simulink model "fuzzy_controller_5_gauss"  (R2016a)
settings: Solver=ode45  StartTime=0.0  StopTime=10.0  RelTol=1e-3
values from neighbouring files (symbols this model uses):
  FORCE_Range_1 = -150    [fuzzy_controller_3_trimf_params.m]    (also in fuzzy_controller_5_gauss_params.m; fuzzy_controller_5_gbell_params.m; fuzzy_controller_5_trimf_optimal_params.m; fuzzy_controller_5_trimf_params.m)
  FORCE_Range_2 = 150    [fuzzy_controller_3_trimf_params.m]    (also in fuzzy_controller_5_gauss_params.m; fuzzy_controller_5_gbell_params.m; fuzzy_controller_5_trimf_optimal_params.m; fuzzy_controller_5_trimf_params.m)
undefined symbols (not defined in the file): fi_1_mu, fi_1_sigma, fi_2_mu, fi_2_sigma, fi_3_mu, fi_3_sigma, fi_4_mu, fi_4_sigma, fi_5_mu, fi_5_sigma, force_1_mu, force_1_sigma, force_2_mu, force_2_sigma, force_3_mu, force_3_sigma, force_4_mu, force_4_sigma, force_5_mu, force_5_sigma, omega_1_mu, omega_1_sigma, omega_2_mu, omega_2_sigma, omega_3_mu, omega_3_sigma, omega_4_mu, omega_4_sigma, omega_5_mu, omega_5_sigma
libraries: fuzwiz x2
settings Model: Creator=Руслан  LastModifiedBy=Руслан
settings DataIOCC: LimitDataPoints=on  SaveFormat=Array
settings DebuggingCC: AlgebraicLoopMsg=error
settings HardwareCC: ProdBitPerLong=64  ProdLargestAtomicFloat=None  ProdHWDeviceType=Intel->x86-64
settings ModelReferenceCC: PropagateSignalLabelsOutOfModel=off
settings RTWCC: TemplateMakefile=RTW.MSVCBuild  Description=Create Visual C/C++ Solution File for Simulink Coder  GenerateReport=on  RetainRTWFile=on  LaunchReport=on
settings CodeAppCC: ForceParamTrailComments=on  MATLABSourceComments=on
settings GRTTargetCC: TargetLangStandard=C99 (ISO)
settings ConfigComp: CovModelRefEnable=Off

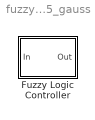
== system fuzzy_controller_5_gauss ==
  Fuzzy Logic Controller : Subsystem

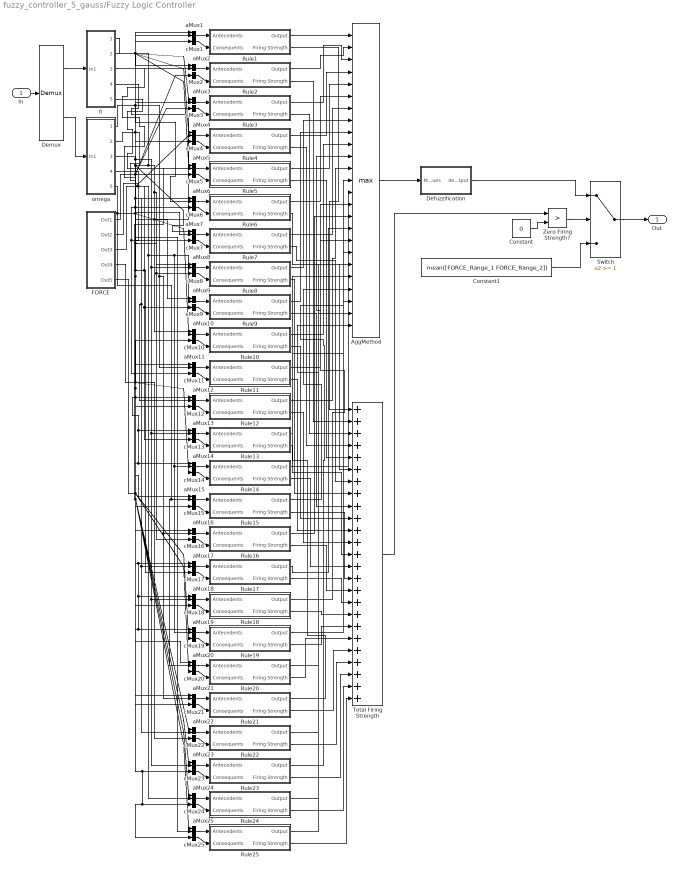
== system fuzzy_controller_5_gauss/Fuzzy Logic Controller ==
  In : Inport
  AggMethod : MinMax  Function=max  Inputs=25
  Constant : Constant  Value=0
  Constant1 : Constant  Value=mean([FORCE_Range_1 FORCE_Range_2])
  Defuzzification : Subsystem
  Demux : Demux  Outputs=2
  FORCE : Subsystem
  Rule1 : Subsystem
  Rule10 : Subsystem
  Rule11 : Subsystem
  Rule12 : Subsystem
  Rule13 : Subsystem
  Rule14 : Subsystem
  Rule15 : Subsystem
  Rule16 : Subsystem
  Rule17 : Subsystem
  Rule18 : Subsystem
  Rule19 : Subsystem
  Rule2 : Subsystem
  Rule20 : Subsystem
  Rule21 : Subsystem
  Rule22 : Subsystem
  Rule23 : Subsystem
  Rule24 : Subsystem
  Rule25 : Subsystem
  Rule3 : Subsystem
  Rule4 : Subsystem
  Rule5 : Subsystem
  Rule6 : Subsystem
  Rule7 : Subsystem
  Rule8 : Subsystem
  Rule9 : Subsystem
  Switch : Switch  Threshold=1
  Total Firing Strength : Sum  Inputs=25
  Zero Firing Strength? : RelationalOperator  Operator=>  OutDataTypeStr=boolean
  aMux{1..25} (25 alike) : Mux  Inputs=2
  cMux{1..25} (25 alike) : Mux  Inputs=1
  fi : Subsystem
  omega : Subsystem
  Out : Outport
  wires:
  Rule1/1(Output) -> AggMethod/1
  Rule2/1(Output) -> AggMethod/2
  Rule5/1(Output) -> AggMethod/5
  Rule4/1(Output) -> AggMethod/4
  Rule3/1(Output) -> AggMethod/3
  Rule1/2(Firing Strength) -> Total Firing Strength/1
  Rule2/2(Firing Strength) -> Total Firing Strength/2
  Rule3/2(Firing Strength) -> Total Firing Strength/3
  Rule4/2(Firing Strength) -> Total Firing Strength/4
  Rule5/2(Firing Strength) -> Total Firing Strength/5
  Total Firing Strength/1 -> Zero Firing Strength?/1
  Constant/1 -> Zero Firing Strength?/2
  Zero Firing Strength?/1 -> Switch/2
  Switch/1 -> Out/1
  Constant1/1 -> Switch/3
  AggMethod/1 -> Defuzzification/1(MF values)
  Defuzzification/1(defuzzified output) -> Switch/1
  Demux/1 -> fi/1(In1)
  In/1 -> Demux/1
  Demux/2 -> omega/1(In1)
  Rule9/2(Firing Strength) -> Total Firing Strength/9
  Rule8/2(Firing Strength) -> Total Firing Strength/8
  Rule7/2(Firing Strength) -> Total Firing Strength/7
  Rule6/2(Firing Strength) -> Total Firing Strength/6
  Rule9/1(Output) -> AggMethod/9
  Rule8/1(Output) -> AggMethod/8
  Rule7/1(Output) -> AggMethod/7
  Rule6/1(Output) -> AggMethod/6
  aMux9/1 -> Rule9/1(Antecedents)
  aMux8/1 -> Rule8/1(Antecedents)
  aMux7/1 -> Rule7/1(Antecedents)
  aMux6/1 -> Rule6/1(Antecedents)
  aMux5/1 -> Rule5/1(Antecedents)
  aMux4/1 -> Rule4/1(Antecedents)
  aMux3/1 -> Rule3/1(Antecedents)
  aMux2/1 -> Rule2/1(Antecedents)
  aMux1/1 -> Rule1/1(Antecedents)
  aMux10/1 -> Rule10/1(Antecedents)
  aMux11/1 -> Rule11/1(Antecedents)
  aMux12/1 -> Rule12/1(Antecedents)
  aMux13/1 -> Rule13/1(Antecedents)
  aMux14/1 -> Rule14/1(Antecedents)
  aMux15/1 -> Rule15/1(Antecedents)
  aMux16/1 -> Rule16/1(Antecedents)
  aMux17/1 -> Rule17/1(Antecedents)
  aMux18/1 -> Rule18/1(Antecedents)
  aMux19/1 -> Rule19/1(Antecedents)
  aMux25/1 -> Rule25/1(Antecedents)
  aMux24/1 -> Rule24/1(Antecedents)
  aMux23/1 -> Rule23/1(Antecedents)
  aMux22/1 -> Rule22/1(Antecedents)
  aMux21/1 -> Rule21/1(Antecedents)
  aMux20/1 -> Rule20/1(Antecedents)
  Rule25/2(Firing Strength) -> Total Firing Strength/25
  Rule10/2(Firing Strength) -> Total Firing Strength/10
  Rule11/2(Firing Strength) -> Total Firing Strength/11
  Rule12/2(Firing Strength) -> Total Firing Strength/12
  Rule13/2(Firing Strength) -> Total Firing Strength/13
  Rule14/2(Firing Strength) -> Total Firing Strength/14
  Rule15/2(Firing Strength) -> Total Firing Strength/15
  Rule16/2(Firing Strength) -> Total Firing Strength/16
  Rule17/2(Firing Strength) -> Total Firing Strength/17
  Rule18/2(Firing Strength) -> Total Firing Strength/18
  Rule19/2(Firing Strength) -> Total Firing Strength/19
  Rule20/2(Firing Strength) -> Total Firing Strength/20
  Rule21/2(Firing Strength) -> Total Firing Strength/21
  Rule22/2(Firing Strength) -> Total Firing Strength/22
  Rule23/2(Firing Strength) -> Total Firing Strength/23
  Rule24/2(Firing Strength) -> Total Firing Strength/24
  Rule10/1(Output) -> AggMethod/10
  Rule11/1(Output) -> AggMethod/11
  Rule12/1(Output) -> AggMethod/12
  Rule13/1(Output) -> AggMethod/13
  Rule14/1(Output) -> AggMethod/14
  Rule15/1(Output) -> AggMethod/15
  Rule16/1(Output) -> AggMethod/16
  Rule25/1(Output) -> AggMethod/25
  Rule17/1(Output) -> AggMethod/17
  Rule18/1(Output) -> AggMethod/18
  Rule19/1(Output) -> AggMethod/19
  Rule20/1(Output) -> AggMethod/20
  Rule21/1(Output) -> AggMethod/21
  Rule22/1(Output) -> AggMethod/22
  Rule23/1(Output) -> AggMethod/23
  Rule24/1(Output) -> AggMethod/24
  cMux1/1 -> Rule1/2(Consequents)
  fi/1(Out1) -> aMux1/1, aMux2/1, aMux3/1, aMux4/1, aMux5/1
  omega/1(Out1) -> aMux16/2, aMux21/2, aMux11/2, aMux1/2, aMux6/2
  FORCE/1(Out1) -> cMux7/1, cMux11/1, cMux6/1, cMux1/1, cMux2/1, cMux3/1
  cMux2/1 -> Rule2/2(Consequents)
  omega/2(Out2) -> aMux7/2, aMux12/2, aMux17/2, aMux22/2, aMux2/2
  cMux3/1 -> Rule3/2(Consequents)
  omega/3(Out3) -> aMux23/2, aMux18/2, aMux13/2, aMux8/2, aMux3/2
  cMux4/1 -> Rule4/2(Consequents)
  omega/4(Out4) -> aMux14/2, aMux19/2, aMux9/2, aMux24/2, aMux4/2
  FORCE/2(Out2) -> cMux8/1, cMux16/1, cMux4/1, cMux12/1
  cMux5/1 -> Rule5/2(Consequents)
  omega/5(Out5) -> aMux5/2, aMux10/2, aMux25/2, aMux20/2, aMux15/2
  FORCE/3(Out3) -> cMux5/1, cMux21/1, cMux17/1, cMux9/1, cMux13/1
  cMux6/1 -> Rule6/2(Consequents)
  fi/2(Out2) -> aMux8/1, aMux9/1, aMux10/1, aMux6/1, aMux7/1
  cMux7/1 -> Rule7/2(Consequents)
  cMux8/1 -> Rule8/2(Consequents)
  cMux9/1 -> Rule9/2(Consequents)
  cMux10/1 -> Rule10/2(Consequents)
  FORCE/4(Out4) -> cMux10/1, cMux14/1, cMux18/1, cMux22/1
  cMux11/1 -> Rule11/2(Consequents)
  fi/3(Out3) -> aMux15/1, aMux14/1, aMux13/1, aMux12/1, aMux11/1
  cMux12/1 -> Rule12/2(Consequents)
  cMux13/1 -> Rule13/2(Consequents)
  cMux14/1 -> Rule14/2(Consequents)
  cMux15/1 -> Rule15/2(Consequents)
  FORCE/5(Out5) -> cMux25/1, cMux24/1, cMux23/1, cMux15/1, cMux19/1, cMux20/1
  cMux16/1 -> Rule16/2(Consequents)
  fi/4(Out4) -> aMux20/1, aMux19/1, aMux18/1, aMux17/1, aMux16/1
  cMux17/1 -> Rule17/2(Consequents)
  cMux18/1 -> Rule18/2(Consequents)
  cMux19/1 -> Rule19/2(Consequents)
  cMux20/1 -> Rule20/2(Consequents)
  cMux21/1 -> Rule21/2(Consequents)
  fi/5(Out5) -> aMux21/1, aMux22/1, aMux23/1, aMux24/1, aMux25/1
  cMux22/1 -> Rule22/2(Consequents)
  cMux23/1 -> Rule23/2(Consequents)
  cMux24/1 -> Rule24/2(Consequents)
  cMux25/1 -> Rule25/2(Consequents)

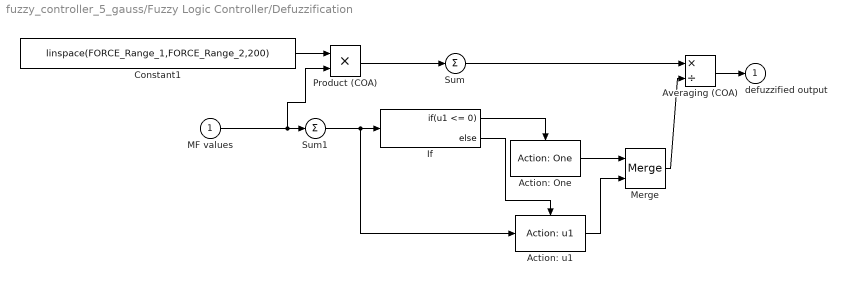
== system fuzzy_controller_5_gauss/Fuzzy Logic Controller/Defuzzification ==
  MF values : Inport
  Action: One : fuzwiz/Centroid of Area/Action: One
  Action: u1 : fuzwiz/Centroid of Area/Action: u1
  Averaging (COA) : Product  Inputs=*/  SaturateOnIntegerOverflow=on  RndMeth=Zero  InputSameDT=on  OutDataTypeStr=Inherit: Same as first input
  Constant1 : Constant  Value=linspace(FORCE_Range_1,FORCE_Range_2,200)
  If : If  IfExpression=u1 <= 0
  Merge : Merge
  Product (COA) : Product  SaturateOnIntegerOverflow=on  RndMeth=Zero  InputSameDT=on  OutDataTypeStr=Inherit: Same as first input
  Sum : Sum  Inputs=+  SaturateOnIntegerOverflow=on  InputSameDT=on  OutDataTypeStr=Inherit: Same as first input
  Sum1 : Sum  Inputs=+  SaturateOnIntegerOverflow=on  InputSameDT=on  OutDataTypeStr=Inherit: Same as first input
  defuzzified output : Outport
  wires:
  Merge/1 -> Averaging (COA)/2
  Action: u1/1 -> Merge/2
  Action: One/1 -> Merge/1
  If/1 -> Action: One/Action
  If/2 -> Action: u1/Action
  Sum1/1 -> Action: u1/1, If/1
  Constant1/1 -> Product (COA)/1
  Product (COA)/1 -> Sum/1
  MF values/1 -> Product (COA)/2, Sum1/1
  Sum/1 -> Averaging (COA)/1
  Averaging (COA)/1 -> defuzzified output/1

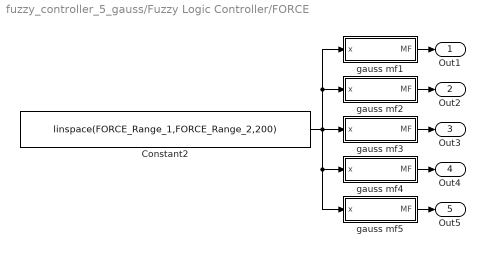
== system fuzzy_controller_5_gauss/Fuzzy Logic Controller/FORCE ==
  Constant2 : Constant  Value=linspace(FORCE_Range_1,FORCE_Range_2,200)
  gauss mf1 : Subsystem  mask{sigma=force_1_sigma, mu=force_1_mu}
      mask prompts: sigma "Variance sigma:"; mu "Mean c:"
  gauss mf2 : Subsystem  mask{sigma=force_2_sigma, mu=force_2_mu}
      mask prompts: sigma "Variance sigma:"; mu "Mean c:"
  gauss mf3 : Subsystem  mask{sigma=force_3_sigma, mu=force_3_mu}
      mask prompts: sigma "Variance sigma:"; mu "Mean c:"
  gauss mf4 : Subsystem  mask{sigma=force_4_sigma, mu=force_4_mu}
      mask prompts: sigma "Variance sigma:"; mu "Mean c:"
  gauss mf5 : Subsystem  mask{sigma=force_5_sigma, mu=force_5_mu}
      mask prompts: sigma "Variance sigma:"; mu "Mean c:"
  Out1 : Outport
  Out2 : Outport  Port=2
  Out3 : Outport  Port=3
  Out4 : Outport  Port=4
  Out5 : Outport  Port=5
  wires:
  Constant2/1 -> gauss mf3/1(x), gauss mf5/1(x), gauss mf4/1(x), gauss mf2/1(x), gauss mf1/1(x)
  gauss mf1/1(MF) -> Out1/1
  gauss mf2/1(MF) -> Out2/1
  gauss mf3/1(MF) -> Out3/1
  gauss mf4/1(MF) -> Out4/1
  gauss mf5/1(MF) -> Out5/1

== system fuzzy_controller_5_gauss/Fuzzy Logic Controller/Rule1 ==
  Antecedents : Inport
  Consequents : Inport  Port=2
  Weight : Constant
  Weighting : Product  SaturateOnIntegerOverflow=on  RndMeth=Zero  InputSameDT=on  OutDataTypeStr=Inherit: Same as first input
  andorMethod : MinMax  SaturateOnIntegerOverflow=on  InputSameDT=on
  impMethod : MinMax  Inputs=2  SaturateOnIntegerOverflow=on  InputSameDT=on
  Output : Outport
  Firing Strength : Outport  Port=2
  wires:
  impMethod/1 -> Output/1
  Weighting/1 -> Firing Strength/1, impMethod/1
  Consequents/1 -> impMethod/2
  Weight/1 -> Weighting/1
  andorMethod/1 -> Weighting/2
  Antecedents/1 -> andorMethod/1

== system fuzzy_controller_5_gauss/Fuzzy Logic Controller/Rule10 ==
  Antecedents : Inport
  Consequents : Inport  Port=2
  Weight : Constant
  Weighting : Product  SaturateOnIntegerOverflow=on  RndMeth=Zero  InputSameDT=on  OutDataTypeStr=Inherit: Same as first input
  andorMethod : MinMax  SaturateOnIntegerOverflow=on  InputSameDT=on
  impMethod : MinMax  Inputs=2  SaturateOnIntegerOverflow=on  InputSameDT=on
  Output : Outport
  Firing Strength : Outport  Port=2
  wires:
  impMethod/1 -> Output/1
  Weighting/1 -> Firing Strength/1, impMethod/1
  Consequents/1 -> impMethod/2
  Weight/1 -> Weighting/1
  andorMethod/1 -> Weighting/2
  Antecedents/1 -> andorMethod/1

== system fuzzy_controller_5_gauss/Fuzzy Logic Controller/Rule11 ==
  Antecedents : Inport
  Consequents : Inport  Port=2
  Weight : Constant
  Weighting : Product  SaturateOnIntegerOverflow=on  RndMeth=Zero  InputSameDT=on  OutDataTypeStr=Inherit: Same as first input
  andorMethod : MinMax  SaturateOnIntegerOverflow=on  InputSameDT=on
  impMethod : MinMax  Inputs=2  SaturateOnIntegerOverflow=on  InputSameDT=on
  Output : Outport
  Firing Strength : Outport  Port=2
  wires:
  impMethod/1 -> Output/1
  Weighting/1 -> Firing Strength/1, impMethod/1
  Consequents/1 -> impMethod/2
  Weight/1 -> Weighting/1
  andorMethod/1 -> Weighting/2
  Antecedents/1 -> andorMethod/1

== system fuzzy_controller_5_gauss/Fuzzy Logic Controller/Rule12 ==
  Antecedents : Inport
  Consequents : Inport  Port=2
  Weight : Constant
  Weighting : Product  SaturateOnIntegerOverflow=on  RndMeth=Zero  InputSameDT=on  OutDataTypeStr=Inherit: Same as first input
  andorMethod : MinMax  SaturateOnIntegerOverflow=on  InputSameDT=on
  impMethod : MinMax  Inputs=2  SaturateOnIntegerOverflow=on  InputSameDT=on
  Output : Outport
  Firing Strength : Outport  Port=2
  wires:
  impMethod/1 -> Output/1
  Weighting/1 -> Firing Strength/1, impMethod/1
  Consequents/1 -> impMethod/2
  Weight/1 -> Weighting/1
  andorMethod/1 -> Weighting/2
  Antecedents/1 -> andorMethod/1

== system fuzzy_controller_5_gauss/Fuzzy Logic Controller/Rule13 ==
  Antecedents : Inport
  Consequents : Inport  Port=2
  Weight : Constant
  Weighting : Product  SaturateOnIntegerOverflow=on  RndMeth=Zero  InputSameDT=on  OutDataTypeStr=Inherit: Same as first input
  andorMethod : MinMax  SaturateOnIntegerOverflow=on  InputSameDT=on
  impMethod : MinMax  Inputs=2  SaturateOnIntegerOverflow=on  InputSameDT=on
  Output : Outport
  Firing Strength : Outport  Port=2
  wires:
  impMethod/1 -> Output/1
  Weighting/1 -> Firing Strength/1, impMethod/1
  Consequents/1 -> impMethod/2
  Weight/1 -> Weighting/1
  andorMethod/1 -> Weighting/2
  Antecedents/1 -> andorMethod/1

== system fuzzy_controller_5_gauss/Fuzzy Logic Controller/Rule14 ==
  Antecedents : Inport
  Consequents : Inport  Port=2
  Weight : Constant
  Weighting : Product  SaturateOnIntegerOverflow=on  RndMeth=Zero  InputSameDT=on  OutDataTypeStr=Inherit: Same as first input
  andorMethod : MinMax  SaturateOnIntegerOverflow=on  InputSameDT=on
  impMethod : MinMax  Inputs=2  SaturateOnIntegerOverflow=on  InputSameDT=on
  Output : Outport
  Firing Strength : Outport  Port=2
  wires:
  impMethod/1 -> Output/1
  Weighting/1 -> Firing Strength/1, impMethod/1
  Consequents/1 -> impMethod/2
  Weight/1 -> Weighting/1
  andorMethod/1 -> Weighting/2
  Antecedents/1 -> andorMethod/1

== system fuzzy_controller_5_gauss/Fuzzy Logic Controller/Rule15 ==
  Antecedents : Inport
  Consequents : Inport  Port=2
  Weight : Constant
  Weighting : Product  SaturateOnIntegerOverflow=on  RndMeth=Zero  InputSameDT=on  OutDataTypeStr=Inherit: Same as first input
  andorMethod : MinMax  SaturateOnIntegerOverflow=on  InputSameDT=on
  impMethod : MinMax  Inputs=2  SaturateOnIntegerOverflow=on  InputSameDT=on
  Output : Outport
  Firing Strength : Outport  Port=2
  wires:
  impMethod/1 -> Output/1
  Weighting/1 -> Firing Strength/1, impMethod/1
  Consequents/1 -> impMethod/2
  Weight/1 -> Weighting/1
  andorMethod/1 -> Weighting/2
  Antecedents/1 -> andorMethod/1

== system fuzzy_controller_5_gauss/Fuzzy Logic Controller/Rule16 ==
  Antecedents : Inport
  Consequents : Inport  Port=2
  Weight : Constant
  Weighting : Product  SaturateOnIntegerOverflow=on  RndMeth=Zero  InputSameDT=on  OutDataTypeStr=Inherit: Same as first input
  andorMethod : MinMax  SaturateOnIntegerOverflow=on  InputSameDT=on
  impMethod : MinMax  Inputs=2  SaturateOnIntegerOverflow=on  InputSameDT=on
  Output : Outport
  Firing Strength : Outport  Port=2
  wires:
  impMethod/1 -> Output/1
  Weighting/1 -> Firing Strength/1, impMethod/1
  Consequents/1 -> impMethod/2
  Weight/1 -> Weighting/1
  andorMethod/1 -> Weighting/2
  Antecedents/1 -> andorMethod/1

== system fuzzy_controller_5_gauss/Fuzzy Logic Controller/Rule17 ==
  Antecedents : Inport
  Consequents : Inport  Port=2
  Weight : Constant
  Weighting : Product  SaturateOnIntegerOverflow=on  RndMeth=Zero  InputSameDT=on  OutDataTypeStr=Inherit: Same as first input
  andorMethod : MinMax  SaturateOnIntegerOverflow=on  InputSameDT=on
  impMethod : MinMax  Inputs=2  SaturateOnIntegerOverflow=on  InputSameDT=on
  Output : Outport
  Firing Strength : Outport  Port=2
  wires:
  impMethod/1 -> Output/1
  Weighting/1 -> Firing Strength/1, impMethod/1
  Consequents/1 -> impMethod/2
  Weight/1 -> Weighting/1
  andorMethod/1 -> Weighting/2
  Antecedents/1 -> andorMethod/1

== system fuzzy_controller_5_gauss/Fuzzy Logic Controller/Rule18 ==
  Antecedents : Inport
  Consequents : Inport  Port=2
  Weight : Constant
  Weighting : Product  SaturateOnIntegerOverflow=on  RndMeth=Zero  InputSameDT=on  OutDataTypeStr=Inherit: Same as first input
  andorMethod : MinMax  SaturateOnIntegerOverflow=on  InputSameDT=on
  impMethod : MinMax  Inputs=2  SaturateOnIntegerOverflow=on  InputSameDT=on
  Output : Outport
  Firing Strength : Outport  Port=2
  wires:
  impMethod/1 -> Output/1
  Weighting/1 -> Firing Strength/1, impMethod/1
  Consequents/1 -> impMethod/2
  Weight/1 -> Weighting/1
  andorMethod/1 -> Weighting/2
  Antecedents/1 -> andorMethod/1

== system fuzzy_controller_5_gauss/Fuzzy Logic Controller/Rule19 ==
  Antecedents : Inport
  Consequents : Inport  Port=2
  Weight : Constant
  Weighting : Product  SaturateOnIntegerOverflow=on  RndMeth=Zero  InputSameDT=on  OutDataTypeStr=Inherit: Same as first input
  andorMethod : MinMax  SaturateOnIntegerOverflow=on  InputSameDT=on
  impMethod : MinMax  Inputs=2  SaturateOnIntegerOverflow=on  InputSameDT=on
  Output : Outport
  Firing Strength : Outport  Port=2
  wires:
  impMethod/1 -> Output/1
  Weighting/1 -> Firing Strength/1, impMethod/1
  Consequents/1 -> impMethod/2
  Weight/1 -> Weighting/1
  andorMethod/1 -> Weighting/2
  Antecedents/1 -> andorMethod/1

== system fuzzy_controller_5_gauss/Fuzzy Logic Controller/Rule2 ==
  Antecedents : Inport
  Consequents : Inport  Port=2
  Weight : Constant
  Weighting : Product  SaturateOnIntegerOverflow=on  RndMeth=Zero  InputSameDT=on  OutDataTypeStr=Inherit: Same as first input
  andorMethod : MinMax  SaturateOnIntegerOverflow=on  InputSameDT=on
  impMethod : MinMax  Inputs=2  SaturateOnIntegerOverflow=on  InputSameDT=on
  Output : Outport
  Firing Strength : Outport  Port=2
  wires:
  impMethod/1 -> Output/1
  Weighting/1 -> Firing Strength/1, impMethod/1
  Consequents/1 -> impMethod/2
  Weight/1 -> Weighting/1
  andorMethod/1 -> Weighting/2
  Antecedents/1 -> andorMethod/1

== system fuzzy_controller_5_gauss/Fuzzy Logic Controller/Rule20 ==
  Antecedents : Inport
  Consequents : Inport  Port=2
  Weight : Constant
  Weighting : Product  SaturateOnIntegerOverflow=on  RndMeth=Zero  InputSameDT=on  OutDataTypeStr=Inherit: Same as first input
  andorMethod : MinMax  SaturateOnIntegerOverflow=on  InputSameDT=on
  impMethod : MinMax  Inputs=2  SaturateOnIntegerOverflow=on  InputSameDT=on
  Output : Outport
  Firing Strength : Outport  Port=2
  wires:
  impMethod/1 -> Output/1
  Weighting/1 -> Firing Strength/1, impMethod/1
  Consequents/1 -> impMethod/2
  Weight/1 -> Weighting/1
  andorMethod/1 -> Weighting/2
  Antecedents/1 -> andorMethod/1

== system fuzzy_controller_5_gauss/Fuzzy Logic Controller/Rule21 ==
  Antecedents : Inport
  Consequents : Inport  Port=2
  Weight : Constant
  Weighting : Product  SaturateOnIntegerOverflow=on  RndMeth=Zero  InputSameDT=on  OutDataTypeStr=Inherit: Same as first input
  andorMethod : MinMax  SaturateOnIntegerOverflow=on  InputSameDT=on
  impMethod : MinMax  Inputs=2  SaturateOnIntegerOverflow=on  InputSameDT=on
  Output : Outport
  Firing Strength : Outport  Port=2
  wires:
  impMethod/1 -> Output/1
  Weighting/1 -> Firing Strength/1, impMethod/1
  Consequents/1 -> impMethod/2
  Weight/1 -> Weighting/1
  andorMethod/1 -> Weighting/2
  Antecedents/1 -> andorMethod/1

== system fuzzy_controller_5_gauss/Fuzzy Logic Controller/Rule22 ==
  Antecedents : Inport
  Consequents : Inport  Port=2
  Weight : Constant
  Weighting : Product  SaturateOnIntegerOverflow=on  RndMeth=Zero  InputSameDT=on  OutDataTypeStr=Inherit: Same as first input
  andorMethod : MinMax  SaturateOnIntegerOverflow=on  InputSameDT=on
  impMethod : MinMax  Inputs=2  SaturateOnIntegerOverflow=on  InputSameDT=on
  Output : Outport
  Firing Strength : Outport  Port=2
  wires:
  impMethod/1 -> Output/1
  Weighting/1 -> Firing Strength/1, impMethod/1
  Consequents/1 -> impMethod/2
  Weight/1 -> Weighting/1
  andorMethod/1 -> Weighting/2
  Antecedents/1 -> andorMethod/1

== system fuzzy_controller_5_gauss/Fuzzy Logic Controller/Rule23 ==
  Antecedents : Inport
  Consequents : Inport  Port=2
  Weight : Constant
  Weighting : Product  SaturateOnIntegerOverflow=on  RndMeth=Zero  InputSameDT=on  OutDataTypeStr=Inherit: Same as first input
  andorMethod : MinMax  SaturateOnIntegerOverflow=on  InputSameDT=on
  impMethod : MinMax  Inputs=2  SaturateOnIntegerOverflow=on  InputSameDT=on
  Output : Outport
  Firing Strength : Outport  Port=2
  wires:
  impMethod/1 -> Output/1
  Weighting/1 -> Firing Strength/1, impMethod/1
  Consequents/1 -> impMethod/2
  Weight/1 -> Weighting/1
  andorMethod/1 -> Weighting/2
  Antecedents/1 -> andorMethod/1

== system fuzzy_controller_5_gauss/Fuzzy Logic Controller/Rule24 ==
  Antecedents : Inport
  Consequents : Inport  Port=2
  Weight : Constant
  Weighting : Product  SaturateOnIntegerOverflow=on  RndMeth=Zero  InputSameDT=on  OutDataTypeStr=Inherit: Same as first input
  andorMethod : MinMax  SaturateOnIntegerOverflow=on  InputSameDT=on
  impMethod : MinMax  Inputs=2  SaturateOnIntegerOverflow=on  InputSameDT=on
  Output : Outport
  Firing Strength : Outport  Port=2
  wires:
  impMethod/1 -> Output/1
  Weighting/1 -> Firing Strength/1, impMethod/1
  Consequents/1 -> impMethod/2
  Weight/1 -> Weighting/1
  andorMethod/1 -> Weighting/2
  Antecedents/1 -> andorMethod/1

== system fuzzy_controller_5_gauss/Fuzzy Logic Controller/Rule25 ==
  Antecedents : Inport
  Consequents : Inport  Port=2
  Weight : Constant
  Weighting : Product  SaturateOnIntegerOverflow=on  RndMeth=Zero  InputSameDT=on  OutDataTypeStr=Inherit: Same as first input
  andorMethod : MinMax  SaturateOnIntegerOverflow=on  InputSameDT=on
  impMethod : MinMax  Inputs=2  SaturateOnIntegerOverflow=on  InputSameDT=on
  Output : Outport
  Firing Strength : Outport  Port=2
  wires:
  impMethod/1 -> Output/1
  Weighting/1 -> Firing Strength/1, impMethod/1
  Consequents/1 -> impMethod/2
  Weight/1 -> Weighting/1
  andorMethod/1 -> Weighting/2
  Antecedents/1 -> andorMethod/1

== system fuzzy_controller_5_gauss/Fuzzy Logic Controller/Rule3 ==
  Antecedents : Inport
  Consequents : Inport  Port=2
  Weight : Constant
  Weighting : Product  SaturateOnIntegerOverflow=on  RndMeth=Zero  InputSameDT=on  OutDataTypeStr=Inherit: Same as first input
  andorMethod : MinMax  SaturateOnIntegerOverflow=on  InputSameDT=on
  impMethod : MinMax  Inputs=2  SaturateOnIntegerOverflow=on  InputSameDT=on
  Output : Outport
  Firing Strength : Outport  Port=2
  wires:
  impMethod/1 -> Output/1
  Weighting/1 -> Firing Strength/1, impMethod/1
  Consequents/1 -> impMethod/2
  Weight/1 -> Weighting/1
  andorMethod/1 -> Weighting/2
  Antecedents/1 -> andorMethod/1

== system fuzzy_controller_5_gauss/Fuzzy Logic Controller/Rule4 ==
  Antecedents : Inport
  Consequents : Inport  Port=2
  Weight : Constant
  Weighting : Product  SaturateOnIntegerOverflow=on  RndMeth=Zero  InputSameDT=on  OutDataTypeStr=Inherit: Same as first input
  andorMethod : MinMax  SaturateOnIntegerOverflow=on  InputSameDT=on
  impMethod : MinMax  Inputs=2  SaturateOnIntegerOverflow=on  InputSameDT=on
  Output : Outport
  Firing Strength : Outport  Port=2
  wires:
  impMethod/1 -> Output/1
  Weighting/1 -> Firing Strength/1, impMethod/1
  Consequents/1 -> impMethod/2
  Weight/1 -> Weighting/1
  andorMethod/1 -> Weighting/2
  Antecedents/1 -> andorMethod/1

== system fuzzy_controller_5_gauss/Fuzzy Logic Controller/Rule5 ==
  Antecedents : Inport
  Consequents : Inport  Port=2
  Weight : Constant
  Weighting : Product  SaturateOnIntegerOverflow=on  RndMeth=Zero  InputSameDT=on  OutDataTypeStr=Inherit: Same as first input
  andorMethod : MinMax  SaturateOnIntegerOverflow=on  InputSameDT=on
  impMethod : MinMax  Inputs=2  SaturateOnIntegerOverflow=on  InputSameDT=on
  Output : Outport
  Firing Strength : Outport  Port=2
  wires:
  impMethod/1 -> Output/1
  Weighting/1 -> Firing Strength/1, impMethod/1
  Consequents/1 -> impMethod/2
  Weight/1 -> Weighting/1
  andorMethod/1 -> Weighting/2
  Antecedents/1 -> andorMethod/1

== system fuzzy_controller_5_gauss/Fuzzy Logic Controller/Rule6 ==
  Antecedents : Inport
  Consequents : Inport  Port=2
  Weight : Constant
  Weighting : Product  SaturateOnIntegerOverflow=on  RndMeth=Zero  InputSameDT=on  OutDataTypeStr=Inherit: Same as first input
  andorMethod : MinMax  SaturateOnIntegerOverflow=on  InputSameDT=on
  impMethod : MinMax  Inputs=2  SaturateOnIntegerOverflow=on  InputSameDT=on
  Output : Outport
  Firing Strength : Outport  Port=2
  wires:
  impMethod/1 -> Output/1
  Weighting/1 -> Firing Strength/1, impMethod/1
  Consequents/1 -> impMethod/2
  Weight/1 -> Weighting/1
  andorMethod/1 -> Weighting/2
  Antecedents/1 -> andorMethod/1

== system fuzzy_controller_5_gauss/Fuzzy Logic Controller/Rule7 ==
  Antecedents : Inport
  Consequents : Inport  Port=2
  Weight : Constant
  Weighting : Product  SaturateOnIntegerOverflow=on  RndMeth=Zero  InputSameDT=on  OutDataTypeStr=Inherit: Same as first input
  andorMethod : MinMax  SaturateOnIntegerOverflow=on  InputSameDT=on
  impMethod : MinMax  Inputs=2  SaturateOnIntegerOverflow=on  InputSameDT=on
  Output : Outport
  Firing Strength : Outport  Port=2
  wires:
  impMethod/1 -> Output/1
  Weighting/1 -> Firing Strength/1, impMethod/1
  Consequents/1 -> impMethod/2
  Weight/1 -> Weighting/1
  andorMethod/1 -> Weighting/2
  Antecedents/1 -> andorMethod/1

== system fuzzy_controller_5_gauss/Fuzzy Logic Controller/Rule8 ==
  Antecedents : Inport
  Consequents : Inport  Port=2
  Weight : Constant
  Weighting : Product  SaturateOnIntegerOverflow=on  RndMeth=Zero  InputSameDT=on  OutDataTypeStr=Inherit: Same as first input
  andorMethod : MinMax  SaturateOnIntegerOverflow=on  InputSameDT=on
  impMethod : MinMax  Inputs=2  SaturateOnIntegerOverflow=on  InputSameDT=on
  Output : Outport
  Firing Strength : Outport  Port=2
  wires:
  impMethod/1 -> Output/1
  Weighting/1 -> Firing Strength/1, impMethod/1
  Consequents/1 -> impMethod/2
  Weight/1 -> Weighting/1
  andorMethod/1 -> Weighting/2
  Antecedents/1 -> andorMethod/1

== system fuzzy_controller_5_gauss/Fuzzy Logic Controller/Rule9 ==
  Antecedents : Inport
  Consequents : Inport  Port=2
  Weight : Constant
  Weighting : Product  SaturateOnIntegerOverflow=on  RndMeth=Zero  InputSameDT=on  OutDataTypeStr=Inherit: Same as first input
  andorMethod : MinMax  SaturateOnIntegerOverflow=on  InputSameDT=on
  impMethod : MinMax  Inputs=2  SaturateOnIntegerOverflow=on  InputSameDT=on
  Output : Outport
  Firing Strength : Outport  Port=2
  wires:
  impMethod/1 -> Output/1
  Weighting/1 -> Firing Strength/1, impMethod/1
  Consequents/1 -> impMethod/2
  Weight/1 -> Weighting/1
  andorMethod/1 -> Weighting/2
  Antecedents/1 -> andorMethod/1

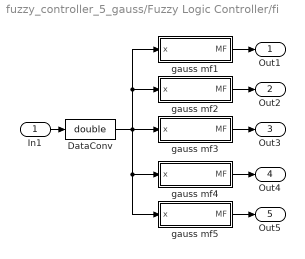
== system fuzzy_controller_5_gauss/Fuzzy Logic Controller/fi ==
  In1 : Inport
  DataConv : DataTypeConversion  OutDataTypeStr=double
  gauss mf1 : Subsystem  mask{sigma=fi_1_sigma, mu=fi_1_mu}
      mask prompts: sigma "Variance sigma:"; mu "Mean c:"
  gauss mf2 : Subsystem  mask{sigma=fi_2_sigma, mu=fi_2_mu}
      mask prompts: sigma "Variance sigma:"; mu "Mean c:"
  gauss mf3 : Subsystem  mask{sigma=fi_3_sigma, mu=fi_3_mu}
      mask prompts: sigma "Variance sigma:"; mu "Mean c:"
  gauss mf4 : Subsystem  mask{sigma=fi_4_sigma, mu=fi_4_mu}
      mask prompts: sigma "Variance sigma:"; mu "Mean c:"
  gauss mf5 : Subsystem  mask{sigma=fi_5_sigma, mu=fi_5_mu}
      mask prompts: sigma "Variance sigma:"; mu "Mean c:"
  Out1 : Outport
  Out2 : Outport  Port=2
  Out3 : Outport  Port=3
  Out4 : Outport  Port=4
  Out5 : Outport  Port=5
  wires:
  In1/1 -> DataConv/1
  gauss mf1/1(MF) -> Out1/1
  gauss mf2/1(MF) -> Out2/1
  gauss mf3/1(MF) -> Out3/1
  DataConv/1 -> gauss mf3/1(x), gauss mf2/1(x), gauss mf1/1(x), gauss mf5/1(x), gauss mf4/1(x)
  gauss mf4/1(MF) -> Out4/1
  gauss mf5/1(MF) -> Out5/1

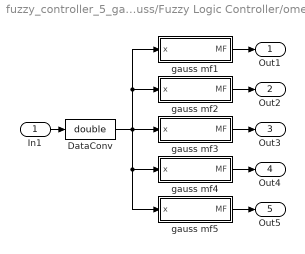
== system fuzzy_controller_5_gauss/Fuzzy Logic Controller/omega ==
  In1 : Inport
  DataConv : DataTypeConversion  OutDataTypeStr=double
  gauss mf1 : Subsystem  mask{sigma=omega_1_sigma, mu=omega_1_mu}
      mask prompts: sigma "Variance sigma:"; mu "Mean c:"
  gauss mf2 : Subsystem  mask{sigma=omega_2_sigma, mu=omega_2_mu}
      mask prompts: sigma "Variance sigma:"; mu "Mean c:"
  gauss mf3 : Subsystem  mask{sigma=omega_3_sigma, mu=omega_3_mu}
      mask prompts: sigma "Variance sigma:"; mu "Mean c:"
  gauss mf4 : Subsystem  mask{sigma=omega_4_sigma, mu=omega_4_mu}
      mask prompts: sigma "Variance sigma:"; mu "Mean c:"
  gauss mf5 : Subsystem  mask{sigma=omega_5_sigma, mu=omega_5_mu}
      mask prompts: sigma "Variance sigma:"; mu "Mean c:"
  Out1 : Outport
  Out2 : Outport  Port=2
  Out3 : Outport  Port=3
  Out4 : Outport  Port=4
  Out5 : Outport  Port=5
  wires:
  In1/1 -> DataConv/1
  gauss mf1/1(MF) -> Out1/1
  gauss mf2/1(MF) -> Out2/1
  gauss mf3/1(MF) -> Out3/1
  DataConv/1 -> gauss mf3/1(x), gauss mf1/1(x), gauss mf2/1(x), gauss mf5/1(x), gauss mf4/1(x)
  gauss mf4/1(MF) -> Out4/1
  gauss mf5/1(MF) -> Out5/1

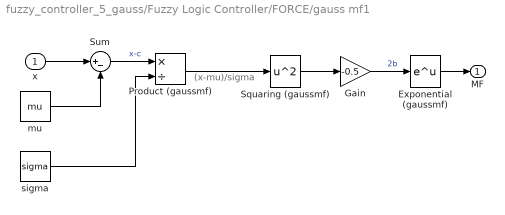
== system fuzzy_controller_5_gauss/Fuzzy Logic Controller/FORCE/gauss mf1 ==
  note: (x-mu)/sigma
  x : Inport
  Exponential (gaussmf) : Math  SaturateOnIntegerOverflow=on
  Gain : Gain  Gain=-0.5  SaturateOnIntegerOverflow=on  OutDataTypeStr=Inherit: Same as input  ParamDataTypeStr=Inherit: Same as input
  Product (gaussmf) : Product  Inputs=*/  SaturateOnIntegerOverflow=on  InputSameDT=on  OutDataTypeStr=Inherit: Same as first input
  Squaring (gaussmf) : Math  Operator=square  SaturateOnIntegerOverflow=on
  Sum : Sum  Inputs=|+-  SaturateOnIntegerOverflow=on  InputSameDT=on  OutDataTypeStr=Inherit: Same as first input
  mu : Constant  Value=mu
  sigma : Constant  Value=sigma
  MF : Outport
  wires:
  Product (gaussmf)/1 -> Squaring (gaussmf)/1
  Gain/1 -> Exponential (gaussmf)/1  "2b"
  Squaring (gaussmf)/1 -> Gain/1
  Exponential (gaussmf)/1 -> MF/1
  sigma/1 -> Product (gaussmf)/2
  Sum/1 -> Product (gaussmf)/1  "x-c"
  mu/1 -> Sum/2
  x/1 -> Sum/1

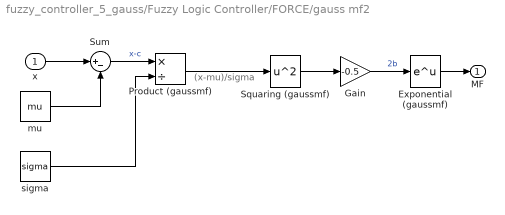
== system fuzzy_controller_5_gauss/Fuzzy Logic Controller/FORCE/gauss mf2 ==
  note: (x-mu)/sigma
  x : Inport
  Exponential (gaussmf) : Math  SaturateOnIntegerOverflow=on
  Gain : Gain  Gain=-0.5  SaturateOnIntegerOverflow=on  OutDataTypeStr=Inherit: Same as input  ParamDataTypeStr=Inherit: Same as input
  Product (gaussmf) : Product  Inputs=*/  SaturateOnIntegerOverflow=on  InputSameDT=on  OutDataTypeStr=Inherit: Same as first input
  Squaring (gaussmf) : Math  Operator=square  SaturateOnIntegerOverflow=on
  Sum : Sum  Inputs=|+-  SaturateOnIntegerOverflow=on  InputSameDT=on  OutDataTypeStr=Inherit: Same as first input
  mu : Constant  Value=mu
  sigma : Constant  Value=sigma
  MF : Outport
  wires:
  Product (gaussmf)/1 -> Squaring (gaussmf)/1
  Gain/1 -> Exponential (gaussmf)/1  "2b"
  Squaring (gaussmf)/1 -> Gain/1
  Exponential (gaussmf)/1 -> MF/1
  sigma/1 -> Product (gaussmf)/2
  Sum/1 -> Product (gaussmf)/1  "x-c"
  mu/1 -> Sum/2
  x/1 -> Sum/1

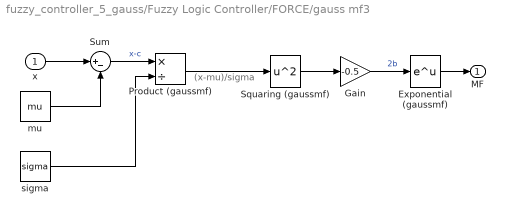
== system fuzzy_controller_5_gauss/Fuzzy Logic Controller/FORCE/gauss mf3 ==
  note: (x-mu)/sigma
  x : Inport
  Exponential (gaussmf) : Math  SaturateOnIntegerOverflow=on
  Gain : Gain  Gain=-0.5  SaturateOnIntegerOverflow=on  OutDataTypeStr=Inherit: Same as input  ParamDataTypeStr=Inherit: Same as input
  Product (gaussmf) : Product  Inputs=*/  SaturateOnIntegerOverflow=on  InputSameDT=on  OutDataTypeStr=Inherit: Same as first input
  Squaring (gaussmf) : Math  Operator=square  SaturateOnIntegerOverflow=on
  Sum : Sum  Inputs=|+-  SaturateOnIntegerOverflow=on  InputSameDT=on  OutDataTypeStr=Inherit: Same as first input
  mu : Constant  Value=mu
  sigma : Constant  Value=sigma
  MF : Outport
  wires:
  Product (gaussmf)/1 -> Squaring (gaussmf)/1
  Gain/1 -> Exponential (gaussmf)/1  "2b"
  Squaring (gaussmf)/1 -> Gain/1
  Exponential (gaussmf)/1 -> MF/1
  sigma/1 -> Product (gaussmf)/2
  Sum/1 -> Product (gaussmf)/1  "x-c"
  mu/1 -> Sum/2
  x/1 -> Sum/1

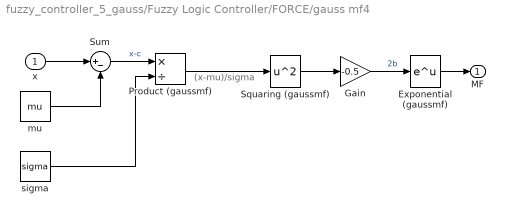
== system fuzzy_controller_5_gauss/Fuzzy Logic Controller/FORCE/gauss mf4 ==
  note: (x-mu)/sigma
  x : Inport
  Exponential (gaussmf) : Math  SaturateOnIntegerOverflow=on
  Gain : Gain  Gain=-0.5  SaturateOnIntegerOverflow=on  OutDataTypeStr=Inherit: Same as input  ParamDataTypeStr=Inherit: Same as input
  Product (gaussmf) : Product  Inputs=*/  SaturateOnIntegerOverflow=on  InputSameDT=on  OutDataTypeStr=Inherit: Same as first input
  Squaring (gaussmf) : Math  Operator=square  SaturateOnIntegerOverflow=on
  Sum : Sum  Inputs=|+-  SaturateOnIntegerOverflow=on  InputSameDT=on  OutDataTypeStr=Inherit: Same as first input
  mu : Constant  Value=mu
  sigma : Constant  Value=sigma
  MF : Outport
  wires:
  Product (gaussmf)/1 -> Squaring (gaussmf)/1
  Gain/1 -> Exponential (gaussmf)/1  "2b"
  Squaring (gaussmf)/1 -> Gain/1
  Exponential (gaussmf)/1 -> MF/1
  sigma/1 -> Product (gaussmf)/2
  Sum/1 -> Product (gaussmf)/1  "x-c"
  mu/1 -> Sum/2
  x/1 -> Sum/1

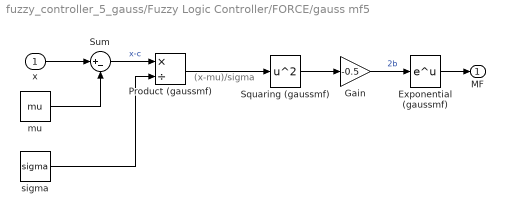
== system fuzzy_controller_5_gauss/Fuzzy Logic Controller/FORCE/gauss mf5 ==
  note: (x-mu)/sigma
  x : Inport
  Exponential (gaussmf) : Math  SaturateOnIntegerOverflow=on
  Gain : Gain  Gain=-0.5  SaturateOnIntegerOverflow=on  OutDataTypeStr=Inherit: Same as input  ParamDataTypeStr=Inherit: Same as input
  Product (gaussmf) : Product  Inputs=*/  SaturateOnIntegerOverflow=on  InputSameDT=on  OutDataTypeStr=Inherit: Same as first input
  Squaring (gaussmf) : Math  Operator=square  SaturateOnIntegerOverflow=on
  Sum : Sum  Inputs=|+-  SaturateOnIntegerOverflow=on  InputSameDT=on  OutDataTypeStr=Inherit: Same as first input
  mu : Constant  Value=mu
  sigma : Constant  Value=sigma
  MF : Outport
  wires:
  Product (gaussmf)/1 -> Squaring (gaussmf)/1
  Gain/1 -> Exponential (gaussmf)/1  "2b"
  Squaring (gaussmf)/1 -> Gain/1
  Exponential (gaussmf)/1 -> MF/1
  sigma/1 -> Product (gaussmf)/2
  Sum/1 -> Product (gaussmf)/1  "x-c"
  mu/1 -> Sum/2
  x/1 -> Sum/1

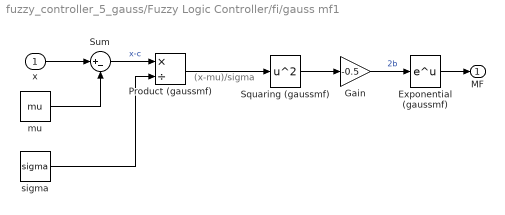
== system fuzzy_controller_5_gauss/Fuzzy Logic Controller/fi/gauss mf1 ==
  note: (x-mu)/sigma
  x : Inport
  Exponential (gaussmf) : Math  SaturateOnIntegerOverflow=on
  Gain : Gain  Gain=-0.5  SaturateOnIntegerOverflow=on  OutDataTypeStr=Inherit: Same as input  ParamDataTypeStr=Inherit: Same as input
  Product (gaussmf) : Product  Inputs=*/  SaturateOnIntegerOverflow=on  InputSameDT=on  OutDataTypeStr=Inherit: Same as first input
  Squaring (gaussmf) : Math  Operator=square  SaturateOnIntegerOverflow=on
  Sum : Sum  Inputs=|+-  SaturateOnIntegerOverflow=on  InputSameDT=on  OutDataTypeStr=Inherit: Same as first input
  mu : Constant  Value=mu
  sigma : Constant  Value=sigma
  MF : Outport
  wires:
  Product (gaussmf)/1 -> Squaring (gaussmf)/1
  Gain/1 -> Exponential (gaussmf)/1  "2b"
  Squaring (gaussmf)/1 -> Gain/1
  Exponential (gaussmf)/1 -> MF/1
  sigma/1 -> Product (gaussmf)/2
  Sum/1 -> Product (gaussmf)/1  "x-c"
  mu/1 -> Sum/2
  x/1 -> Sum/1

== system fuzzy_controller_5_gauss/Fuzzy Logic Controller/fi/gauss mf2 ==
  note: (x-mu)/sigma
  x : Inport
  Exponential (gaussmf) : Math  SaturateOnIntegerOverflow=on
  Gain : Gain  Gain=-0.5  SaturateOnIntegerOverflow=on  OutDataTypeStr=Inherit: Same as input  ParamDataTypeStr=Inherit: Same as input
  Product (gaussmf) : Product  Inputs=*/  SaturateOnIntegerOverflow=on  InputSameDT=on  OutDataTypeStr=Inherit: Same as first input
  Squaring (gaussmf) : Math  Operator=square  SaturateOnIntegerOverflow=on
  Sum : Sum  Inputs=|+-  SaturateOnIntegerOverflow=on  InputSameDT=on  OutDataTypeStr=Inherit: Same as first input
  mu : Constant  Value=mu
  sigma : Constant  Value=sigma
  MF : Outport
  wires:
  Product (gaussmf)/1 -> Squaring (gaussmf)/1
  Gain/1 -> Exponential (gaussmf)/1  "2b"
  Squaring (gaussmf)/1 -> Gain/1
  Exponential (gaussmf)/1 -> MF/1
  sigma/1 -> Product (gaussmf)/2
  Sum/1 -> Product (gaussmf)/1  "x-c"
  mu/1 -> Sum/2
  x/1 -> Sum/1

== system fuzzy_controller_5_gauss/Fuzzy Logic Controller/fi/gauss mf3 ==
  note: (x-mu)/sigma
  x : Inport
  Exponential (gaussmf) : Math  SaturateOnIntegerOverflow=on
  Gain : Gain  Gain=-0.5  SaturateOnIntegerOverflow=on  OutDataTypeStr=Inherit: Same as input  ParamDataTypeStr=Inherit: Same as input
  Product (gaussmf) : Product  Inputs=*/  SaturateOnIntegerOverflow=on  InputSameDT=on  OutDataTypeStr=Inherit: Same as first input
  Squaring (gaussmf) : Math  Operator=square  SaturateOnIntegerOverflow=on
  Sum : Sum  Inputs=|+-  SaturateOnIntegerOverflow=on  InputSameDT=on  OutDataTypeStr=Inherit: Same as first input
  mu : Constant  Value=mu
  sigma : Constant  Value=sigma
  MF : Outport
  wires:
  Product (gaussmf)/1 -> Squaring (gaussmf)/1
  Gain/1 -> Exponential (gaussmf)/1  "2b"
  Squaring (gaussmf)/1 -> Gain/1
  Exponential (gaussmf)/1 -> MF/1
  sigma/1 -> Product (gaussmf)/2
  Sum/1 -> Product (gaussmf)/1  "x-c"
  mu/1 -> Sum/2
  x/1 -> Sum/1

== system fuzzy_controller_5_gauss/Fuzzy Logic Controller/fi/gauss mf4 ==
  note: (x-mu)/sigma
  x : Inport
  Exponential (gaussmf) : Math  SaturateOnIntegerOverflow=on
  Gain : Gain  Gain=-0.5  SaturateOnIntegerOverflow=on  OutDataTypeStr=Inherit: Same as input  ParamDataTypeStr=Inherit: Same as input
  Product (gaussmf) : Product  Inputs=*/  SaturateOnIntegerOverflow=on  InputSameDT=on  OutDataTypeStr=Inherit: Same as first input
  Squaring (gaussmf) : Math  Operator=square  SaturateOnIntegerOverflow=on
  Sum : Sum  Inputs=|+-  SaturateOnIntegerOverflow=on  InputSameDT=on  OutDataTypeStr=Inherit: Same as first input
  mu : Constant  Value=mu
  sigma : Constant  Value=sigma
  MF : Outport
  wires:
  Product (gaussmf)/1 -> Squaring (gaussmf)/1
  Gain/1 -> Exponential (gaussmf)/1  "2b"
  Squaring (gaussmf)/1 -> Gain/1
  Exponential (gaussmf)/1 -> MF/1
  sigma/1 -> Product (gaussmf)/2
  Sum/1 -> Product (gaussmf)/1  "x-c"
  mu/1 -> Sum/2
  x/1 -> Sum/1

== system fuzzy_controller_5_gauss/Fuzzy Logic Controller/fi/gauss mf5 ==
  note: (x-mu)/sigma
  x : Inport
  Exponential (gaussmf) : Math  SaturateOnIntegerOverflow=on
  Gain : Gain  Gain=-0.5  SaturateOnIntegerOverflow=on  OutDataTypeStr=Inherit: Same as input  ParamDataTypeStr=Inherit: Same as input
  Product (gaussmf) : Product  Inputs=*/  SaturateOnIntegerOverflow=on  InputSameDT=on  OutDataTypeStr=Inherit: Same as first input
  Squaring (gaussmf) : Math  Operator=square  SaturateOnIntegerOverflow=on
  Sum : Sum  Inputs=|+-  SaturateOnIntegerOverflow=on  InputSameDT=on  OutDataTypeStr=Inherit: Same as first input
  mu : Constant  Value=mu
  sigma : Constant  Value=sigma
  MF : Outport
  wires:
  Product (gaussmf)/1 -> Squaring (gaussmf)/1
  Gain/1 -> Exponential (gaussmf)/1  "2b"
  Squaring (gaussmf)/1 -> Gain/1
  Exponential (gaussmf)/1 -> MF/1
  sigma/1 -> Product (gaussmf)/2
  Sum/1 -> Product (gaussmf)/1  "x-c"
  mu/1 -> Sum/2
  x/1 -> Sum/1

== system fuzzy_controller_5_gauss/Fuzzy Logic Controller/omega/gauss mf1 ==
  note: (x-mu)/sigma
  x : Inport
  Exponential (gaussmf) : Math  SaturateOnIntegerOverflow=on
  Gain : Gain  Gain=-0.5  SaturateOnIntegerOverflow=on  OutDataTypeStr=Inherit: Same as input  ParamDataTypeStr=Inherit: Same as input
  Product (gaussmf) : Product  Inputs=*/  SaturateOnIntegerOverflow=on  InputSameDT=on  OutDataTypeStr=Inherit: Same as first input
  Squaring (gaussmf) : Math  Operator=square  SaturateOnIntegerOverflow=on
  Sum : Sum  Inputs=|+-  SaturateOnIntegerOverflow=on  InputSameDT=on  OutDataTypeStr=Inherit: Same as first input
  mu : Constant  Value=mu
  sigma : Constant  Value=sigma
  MF : Outport
  wires:
  Product (gaussmf)/1 -> Squaring (gaussmf)/1
  Gain/1 -> Exponential (gaussmf)/1  "2b"
  Squaring (gaussmf)/1 -> Gain/1
  Exponential (gaussmf)/1 -> MF/1
  sigma/1 -> Product (gaussmf)/2
  Sum/1 -> Product (gaussmf)/1  "x-c"
  mu/1 -> Sum/2
  x/1 -> Sum/1

== system fuzzy_controller_5_gauss/Fuzzy Logic Controller/omega/gauss mf2 ==
  note: (x-mu)/sigma
  x : Inport
  Exponential (gaussmf) : Math  SaturateOnIntegerOverflow=on
  Gain : Gain  Gain=-0.5  SaturateOnIntegerOverflow=on  OutDataTypeStr=Inherit: Same as input  ParamDataTypeStr=Inherit: Same as input
  Product (gaussmf) : Product  Inputs=*/  SaturateOnIntegerOverflow=on  InputSameDT=on  OutDataTypeStr=Inherit: Same as first input
  Squaring (gaussmf) : Math  Operator=square  SaturateOnIntegerOverflow=on
  Sum : Sum  Inputs=|+-  SaturateOnIntegerOverflow=on  InputSameDT=on  OutDataTypeStr=Inherit: Same as first input
  mu : Constant  Value=mu
  sigma : Constant  Value=sigma
  MF : Outport
  wires:
  Product (gaussmf)/1 -> Squaring (gaussmf)/1
  Gain/1 -> Exponential (gaussmf)/1  "2b"
  Squaring (gaussmf)/1 -> Gain/1
  Exponential (gaussmf)/1 -> MF/1
  sigma/1 -> Product (gaussmf)/2
  Sum/1 -> Product (gaussmf)/1  "x-c"
  mu/1 -> Sum/2
  x/1 -> Sum/1

== system fuzzy_controller_5_gauss/Fuzzy Logic Controller/omega/gauss mf3 ==
  note: (x-mu)/sigma
  x : Inport
  Exponential (gaussmf) : Math  SaturateOnIntegerOverflow=on
  Gain : Gain  Gain=-0.5  SaturateOnIntegerOverflow=on  OutDataTypeStr=Inherit: Same as input  ParamDataTypeStr=Inherit: Same as input
  Product (gaussmf) : Product  Inputs=*/  SaturateOnIntegerOverflow=on  InputSameDT=on  OutDataTypeStr=Inherit: Same as first input
  Squaring (gaussmf) : Math  Operator=square  SaturateOnIntegerOverflow=on
  Sum : Sum  Inputs=|+-  SaturateOnIntegerOverflow=on  InputSameDT=on  OutDataTypeStr=Inherit: Same as first input
  mu : Constant  Value=mu
  sigma : Constant  Value=sigma
  MF : Outport
  wires:
  Product (gaussmf)/1 -> Squaring (gaussmf)/1
  Gain/1 -> Exponential (gaussmf)/1  "2b"
  Squaring (gaussmf)/1 -> Gain/1
  Exponential (gaussmf)/1 -> MF/1
  sigma/1 -> Product (gaussmf)/2
  Sum/1 -> Product (gaussmf)/1  "x-c"
  mu/1 -> Sum/2
  x/1 -> Sum/1

== system fuzzy_controller_5_gauss/Fuzzy Logic Controller/omega/gauss mf4 ==
  note: (x-mu)/sigma
  x : Inport
  Exponential (gaussmf) : Math  SaturateOnIntegerOverflow=on
  Gain : Gain  Gain=-0.5  SaturateOnIntegerOverflow=on  OutDataTypeStr=Inherit: Same as input  ParamDataTypeStr=Inherit: Same as input
  Product (gaussmf) : Product  Inputs=*/  SaturateOnIntegerOverflow=on  InputSameDT=on  OutDataTypeStr=Inherit: Same as first input
  Squaring (gaussmf) : Math  Operator=square  SaturateOnIntegerOverflow=on
  Sum : Sum  Inputs=|+-  SaturateOnIntegerOverflow=on  InputSameDT=on  OutDataTypeStr=Inherit: Same as first input
  mu : Constant  Value=mu
  sigma : Constant  Value=sigma
  MF : Outport
  wires:
  Product (gaussmf)/1 -> Squaring (gaussmf)/1
  Gain/1 -> Exponential (gaussmf)/1  "2b"
  Squaring (gaussmf)/1 -> Gain/1
  Exponential (gaussmf)/1 -> MF/1
  sigma/1 -> Product (gaussmf)/2
  Sum/1 -> Product (gaussmf)/1  "x-c"
  mu/1 -> Sum/2
  x/1 -> Sum/1

== system fuzzy_controller_5_gauss/Fuzzy Logic Controller/omega/gauss mf5 ==
  note: (x-mu)/sigma
  x : Inport
  Exponential (gaussmf) : Math  SaturateOnIntegerOverflow=on
  Gain : Gain  Gain=-0.5  SaturateOnIntegerOverflow=on  OutDataTypeStr=Inherit: Same as input  ParamDataTypeStr=Inherit: Same as input
  Product (gaussmf) : Product  Inputs=*/  SaturateOnIntegerOverflow=on  InputSameDT=on  OutDataTypeStr=Inherit: Same as first input
  Squaring (gaussmf) : Math  Operator=square  SaturateOnIntegerOverflow=on
  Sum : Sum  Inputs=|+-  SaturateOnIntegerOverflow=on  InputSameDT=on  OutDataTypeStr=Inherit: Same as first input
  mu : Constant  Value=mu
  sigma : Constant  Value=sigma
  MF : Outport
  wires:
  Product (gaussmf)/1 -> Squaring (gaussmf)/1
  Gain/1 -> Exponential (gaussmf)/1  "2b"
  Squaring (gaussmf)/1 -> Gain/1
  Exponential (gaussmf)/1 -> MF/1
  sigma/1 -> Product (gaussmf)/2
  Sum/1 -> Product (gaussmf)/1  "x-c"
  mu/1 -> Sum/2
  x/1 -> Sum/1
